simulink model "sampleModel1739"  (R2022a)
settings: Solver=FixedStepAuto  StartTime=0.0  StopTime=10.0  RelTol=1e-3
undefined symbols (not defined in the file): DiscIntNeverNeededParam, Newton, Raphson
libraries: simulink x34, slpidlib x7
(part 1 of 2)
settings Model: SimulationMode=software-in-the-loop (sil)  Creator=lenovo  LastModifiedBy=TSMC
settings DataIOCC: InspectSignalLogs=on  SignalLoggingName=logsOut
settings OptimizationCC: DefaultParameterBehavior=Inlined  EnhancedBackFolding=on  PassReuseOutputArgsAs=Individual arguments  ZeroExternalMemoryAtStartup=off  ZeroInternalMemoryAtStartup=off  OptimizeBlockOrder=speed  DifferentSizesBufferReuse=on  OptimizationCustomize=off  EfficientTunableParamExpr=on
settings DebuggingCC: ParameterTunabilityLossMsg=error  UnconnectedInputMsg=warning  UnconnectedOutputMsg=warning  UnconnectedLineMsg=warning
settings ModelReferenceCC: UpdateModelReferenceTargets=Force
settings SFSimCC: MATLABDynamicMemAlloc=off
settings RTWCC: SystemTargetFile=ert.tlc  TemplateMakefile=ert_default_tmf  GenerateReport=on  IncludeHyperlinkInReport=on  GenerateTraceInfo=on  DLArmComputeVersion=19.05
settings CodeAppCC: ForceParamTrailComments=on  IgnoreCustomStorageClasses=off  OperatorAnnotations=on  SimulinkDataObjDesc=on  SFDataObjDesc=on  InsertBlockDesc=on
settings ERTTargetCC: TargetLangStandard=C99 (ISO)  GenerateSampleERTMain=on  SupportContinuousTime=on  InlinedParameterPlacement=NonHierarchical  ERTCustomFileTemplate=example_file_process.tlc

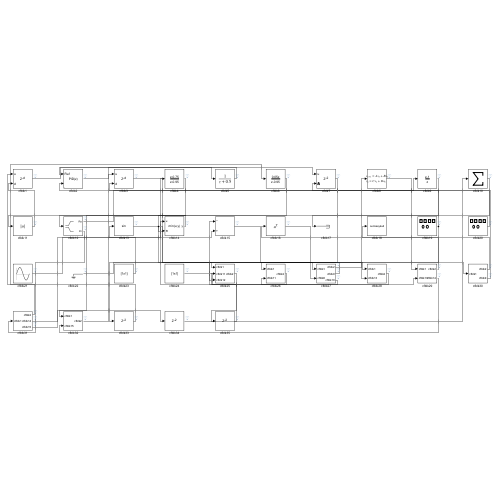
[thumbnail: Simulink's stored preview of the top-level diagram]
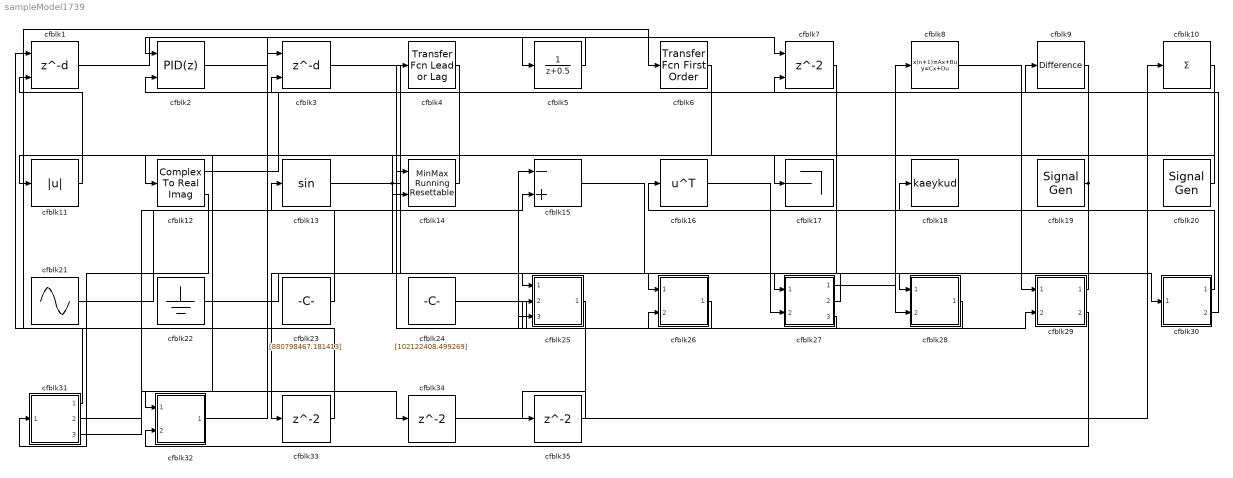
== system sampleModel1739 ==
  cfblk1 : Delay  DelayLengthSource=Input port  SampleTime=1
      settings: InputPortMap=u0,p1
  cfblk10 : Sum  Inputs=+
  cfblk11 : Abs  SaturateOnIntegerOverflow=off
  cfblk12 : ComplexToRealImag
  cfblk13 : Trigonometry
  cfblk14 : simulink/Math Operations/MinMax Running Resettable  Function=min  vinit=0.0
  cfblk15 : Sum  Inputs=-+
  cfblk16 : Math  Operator=transpose
  cfblk17 : Terminator
  cfblk18 : ToWorkspace  VariableName=kaeykud  SaveFormat=Timeseries  SampleTime=-1
  cfblk19 : SignalGenerator  WaveForm=sawtooth  Amplitude=[-934882959.011035]  Units=rad/sec
  cfblk2 : slpidlib/PID Controller (2DOF)  Controller=PID  Form=Parallel  TimeDomain=Discrete-time  UseExternalTs=off  SampleTime=1  IntegratorMethod=Forward Euler  FilterMethod=Forward Euler  ControllerParametersSource=internal  P=1  I=1  UseKiTs=off  D=0  N=100  UseFilter=on  b=1  c=1  TunerSelectOption=Transfer Function Based (PID Tuner App)  InitialConditionSource=internal  InitialConditionForIntegrator=0  InitialConditionForFilter=0  DifferentiatorICPrevScaledInput=0  ExternalReset=none  TrackingMode=off  Kt=1  LimitOutput=off  SatLimitsSource=internal  UpperSaturationLimit=inf  LowerSaturationLimit=-inf  LinearizeAsGain=off  AntiWindupMode=none  Kb=1  POutMin=[]  POutMax=[]  IOutMin=[]  IOutMax=[]  DOutMin=[]  DOutMax=[]  NOutMin=[]  NOutMax=[]  bOutMin=[]  bOutMax=[]  cOutMin=[]  cOutMax=[]  SumOutMin=[]  SumOutMax=[]  SaturationOutMin=[]  SaturationOutMax=[]  PParamMin=[]  PParamMax=[]  IParamMin=[]  IParamMax=[]  DParamMin=[]  DParamMax=[]  NParamMin=[]  NParamMax=[]  bParamMin=[]  bParamMax=[]  cParamMin=[]  cParamMax=[]  KbParamMin=[]  KbParamMax=[]  KtParamMin=[]  KtParamMax=[]  KbOutMin=[]  KbOutMax=[]  KtOutMin=[]  KtOutMax=[]  IntegratorOutMin=[]  IntegratorOutMax=[]  FilterOutMin=[]  FilterOutMax=[]  SumI1OutMin=[]  SumI1OutMax=[]  SumI2OutMin=[]  SumI2OutMax=[]  SumI3OutMin=[]  SumI3OutMax=[]  SumI4OutMin=[]  SumI4OutMax=[]  SumDOutMin=[]  SumDOutMax=[]  Sum1OutMin=[]  Sum1OutMax=[]  Sum2OutMin=[]  Sum2OutMax=[]  Sum3OutMin=[]  Sum3OutMax=[]  DifferentiatorOutMin=[]  DifferentiatorOutMax=[]  FilterDiffOutCoefMin=[]  FilterDiffOutCoefMax=[]  ReciprocalOutMin=[]  ReciprocalOutMax=[]  SumDenOutMin=[]  SumDenOutMax=[]  SumNumOutMin=[]  SumNumOutMax=[]  DivideOutMin=[]  DivideOutMax=[]  UdiffTsProdOutMin=[]  UdiffTsProdOutMax=[]  NTsProdOutMin=[]  NTsProdOutMax=[]  UintegralTsProdOutMin=[]  UintegralTsProdOutMax=[]  UngainTsProdOutMin=[]  UngainTsProdOutMax=[]  IntegratorContinuousStateAttributes=''  IntegratorStateMustResolveToSignalObject=off  IntegratorRTWStateStorageClass=Auto  FilterContinuousStateAttributes=''  FilterStateMustResolveToSignalObject=off  FilterRTWStateStorageClass=Auto  ParallelPVariant=InternalParameters  IdealPVariant=Disabled  IVariant=InternalParameters  DVariant=InternalParameters  bVariant=InternalParameters  cVariant=InternalParameters  IntegratorVariant=Discrete  SatVariant=Disabled  AWVariant=Passthrough  PCopyVariant=Disabled  TRVariant=Disabled  FdbkBlocksVariant=Forward  IdealPFdbkVariant=Disabled  SatFdbkVariant=Disabled  DerivativeFilterVariant=ForwardEulerFilter  NVariant=InternalParameters  NCopyVariant=Disabled  FilterICVariant=InternalICsFilter  IntegratorICVariant=InternalICs  ExternalResetVariant=Disabled  TRSumVariant=Passthrough  SumFdbkVariant=Disabled  SumVariant=Sum_PID  TsampFilterVariant=InternalTs  TsampNgainVariant=Passthrough  TsampIntegralVariant=Passthrough  ExternalSaturationOutDataTypeStr=Inherit: Same as second input
      settings: SourceProductBaseCode=SL
  cfblk20 : SignalGenerator  WaveForm=square  Amplitude=[-890295358.214809]
  cfblk21 : Sin  Amplitude=[-919056267.570477]  Bias=[51069111.724816]  SampleTime=0
  cfblk22 : Ground
  cfblk23 : Constant  Value=[880798467.181413]  SampleTime=1
  cfblk24 : Constant  Value=[102122408.499269]  SampleTime=1
  cfblk25 : Subsystem
  cfblk26 : Subsystem
  cfblk27 : Subsystem
  cfblk28 : Subsystem
  cfblk29 : Subsystem
  cfblk3 : Delay  DelayLengthSource=Input port  SampleTime=1
      settings: InputPortMap=u0,p1
  cfblk30 : Subsystem
  cfblk31 : Subsystem
  cfblk32 : Subsystem
  cfblk33 : Delay  SampleTime=1
  cfblk34 : Delay  SampleTime=1
  cfblk35 : Delay  SampleTime=1
  cfblk4 : simulink/Discrete/Transfer Fcn Lead or Lag  PoleZ=0.95  ZeroZ=0.75  ICPrevOutput=0.0  ICPrevInput=0.0  DoSatur=off
      settings: SourceProductBaseCode=SL
  cfblk5 : DiscreteTransferFcn  SampleTime=1
  cfblk6 : simulink/Discrete/Transfer Fcn First Order  PoleZ=0.95  ICPrevOutput=0.0  DoSatur=off
  cfblk7 : Delay  ShowEnablePort=on  SampleTime=1
      settings: InputPortMap=u0,e6
  cfblk8 : DiscreteStateSpace
  cfblk9 : simulink/Discrete/Difference  ICPrevInput=0.0  OutMin=[]  OutMax=[]  OutDataTypeStr=Inherit: Inherit via back propagation  OutDataType=fixdt(1, 16)  OutScaling=2^-10  DoSatur=off
  wires:
  cfblk30/1(cfblk2) -> cfblk16/1
  cfblk1/1 -> cfblk5/1
  cfblk3/1 -> cfblk30/1(cfblk1)
  cfblk28/1(cfblk2) -> cfblk4/1
  cfblk15/1 -> cfblk27/1(cfblk1)
  cfblk31/1(cfblk2) -> cfblk6/1
  cfblk14/1 -> cfblk12/1
  cfblk23/1 -> cfblk13/1
  cfblk4/1 -> cfblk11/1
  cfblk32/1(cfblk2) -> cfblk3/1
  cfblk13/1 -> cfblk27/2(cfblk8), cfblk28/2(cfblk13)
  cfblk12/1 -> cfblk9/1
  cfblk8/1 -> cfblk29/1(cfblk1)
  cfblk24/1 -> cfblk29/2(cfblk13)
  cfblk12/2 -> cfblk31/1(cfblk1)
  cfblk2/1 -> cfblk7/1
  cfblk9/1 -> cfblk17/1
  cfblk20/1 -> cfblk3/2
  cfblk6/1 -> cfblk32/1(cfblk1)
  cfblk11/1 -> cfblk1/2
  cfblk21/1 -> cfblk14/1
  cfblk5/1 -> cfblk2/1
  cfblk29/1(cfblk2) -> cfblk18/1
  cfblk19/1 -> cfblk2/2, cfblk25/3(cfblk12)
  cfblk31/3(cfblk15) -> cfblk15/2
  cfblk30/2(cfblk9) -> cfblk7/2
  cfblk27/1(cfblk2) -> cfblk8/1
  cfblk10/1 -> cfblk14/2
  cfblk16/1 -> cfblk28/1(cfblk1)
  cfblk22/1 -> cfblk25/1(cfblk1)
  cfblk29/2(cfblk14) -> cfblk32/2(cfblk15)
  cfblk27/2(cfblk9) -> cfblk26/1(cfblk1)
  cfblk27/3(cfblk10) -> cfblk26/2(cfblk11)
  cfblk26/1(cfblk2) -> cfblk25/2(cfblk11)
  cfblk7/1 -> cfblk33/1
  cfblk33/1 -> cfblk1/1
  cfblk31/2(cfblk14) -> cfblk34/1
  cfblk34/1 -> cfblk10/1
  cfblk25/1(cfblk2) -> cfblk35/1
  cfblk35/1 -> cfblk15/1

== system sampleModel1739/cfblk25 ==
  cfblk1 : Inport
  cfblk11 : Inport  Port=2
  cfblk12 : Inport  Port=3
  cfblk10 : Subsystem
  cfblk13 : Delay  SampleTime=1
  cfblk14 : Delay  SampleTime=1
  cfblk3 : simulink/Discrete/Tapped Delay  vinit=0.0  samptime=-1  NumDelays=1  DelayOrder=Oldest  includeCurrent=off
  cfblk4 : Signum
  cfblk5 : Sum
  cfblk6 : Sum  Inputs=+
  cfblk7 : Assignment  DiagnosticForDimensions=Warning  IndexOptions=Index vector (dialog)  Indices=1  OutputSizes=1
  cfblk8 : Constant  Value=[-767685989.889519]  SampleTime=1
  cfblk9 : Subsystem
  cfblk2 : Outport
  wires:
  cfblk10/1(cfblk2) -> cfblk9/1(cfblk1)
  cfblk8/1 -> cfblk3/1
  cfblk12/1 -> cfblk7/1
  cfblk4/1 -> cfblk10/2(cfblk14), cfblk9/4(cfblk9)
  cfblk11/1 -> cfblk10/3(cfblk15)
  cfblk10/2(cfblk17) -> cfblk9/2(cfblk7)
  cfblk5/1 -> cfblk7/2
  cfblk6/1 -> cfblk10/4(cfblk16), cfblk5/1
  cfblk1/1 -> cfblk2/1
  cfblk3/1 -> cfblk6/1, cfblk9/3(cfblk8)
  cfblk7/1 -> cfblk4/1, cfblk14/1
  cfblk9/1(cfblk2) -> cfblk13/1
  cfblk13/1 -> cfblk10/1(cfblk1)
  cfblk14/1 -> cfblk5/2

== system sampleModel1739/cfblk26 ==
  cfblk1 : Inport
  cfblk11 : Inport  Port=2
  cfblk10 : Subsystem
  cfblk12 : Delay  SampleTime=1
  cfblk3 : simulink/Discrete/Transfer Fcn First Order  PoleZ=0.95  ICPrevOutput=0.0  DoSatur=off
  cfblk4 : Sum  Inputs=|++
  cfblk5 : MinMax  Function=max  Inputs=2
  cfblk6 : Sin  TimeSource=Use external signal  SampleTime=0
  cfblk7 : Signum
  cfblk8 : Subsystem
  cfblk9 : Subsystem
  cfblk2 : Outport
  wires:
  cfblk4/1 -> cfblk7/1
  cfblk3/1 -> cfblk4/1, cfblk5/1
  cfblk1/1 -> cfblk10/1(cfblk1)
  cfblk8/1(cfblk2) -> cfblk9/1(cfblk1)
  cfblk11/1 -> cfblk4/2, cfblk8/1(cfblk1)
  cfblk9/1(cfblk2) -> cfblk10/2(cfblk6)
  cfblk10/1(cfblk2) -> cfblk6/1
  cfblk6/1 -> cfblk2/1
  cfblk7/1 -> cfblk9/2(cfblk8), cfblk9/3(cfblk9)
  cfblk9/2(cfblk10) -> cfblk10/3(cfblk7), cfblk5/2
  cfblk5/1 -> cfblk12/1
  cfblk12/1 -> cfblk3/1

== system sampleModel1739/cfblk27 ==
  cfblk1 : Inport
  cfblk8 : Inport  Port=2
  cfblk11 : Delay  SampleTime=1
  cfblk3 : Delay  SampleTime=1
  cfblk4 : DiscreteFilter  SampleTime=1
  cfblk5 : Bias  Bias=[214657201.126867]  SaturateOnIntegerOverflow=off
  cfblk6 : Constant  Value=[682272621.447085]  SampleTime=1
  cfblk7 : Subsystem
  cfblk2 : Outport
  cfblk9 : Outport  Port=2
  cfblk10 : Outport  Port=3
  wires:
  cfblk1/1 -> cfblk2/1
  cfblk8/1 -> cfblk3/1, cfblk7/2(cfblk10)
  cfblk3/1 -> cfblk10/1
  cfblk5/1 -> cfblk4/1, cfblk7/3(cfblk11)
  cfblk4/1 -> cfblk9/1
  cfblk6/1 -> cfblk7/1(cfblk1), cfblk7/4(cfblk12), cfblk7/5(cfblk13)
  cfblk7/1(cfblk2) -> cfblk11/1
  cfblk11/1 -> cfblk5/1

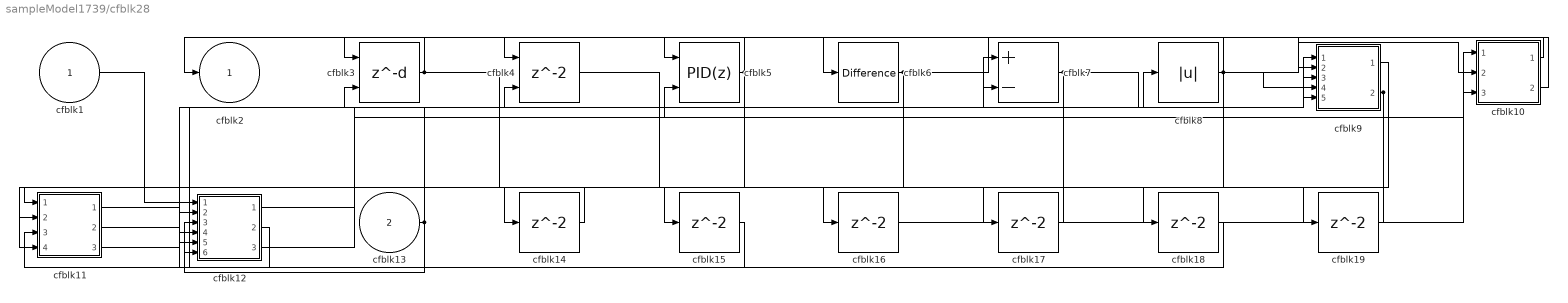
== system sampleModel1739/cfblk28 ==
  cfblk1 : Inport
  cfblk13 : Inport  Port=2
  cfblk10 : Subsystem
  cfblk11 : Subsystem
  cfblk12 : Subsystem
  cfblk{14..19} (6 alike) : Delay  SampleTime=1
  cfblk3 : Delay  DelayLengthSource=Input port  SampleTime=1
      settings: InputPortMap=u0,p1
  cfblk4 : Delay  ShowEnablePort=on  SampleTime=1
      settings: InputPortMap=u0,e6
  cfblk5 : slpidlib/PID Controller (2DOF)  Controller=PID  Form=Parallel  TimeDomain=Discrete-time  UseExternalTs=off  SampleTime=1  IntegratorMethod=Forward Euler  FilterMethod=Forward Euler  ControllerParametersSource=internal  P=1  I=1  UseKiTs=off  D=0  N=100  UseFilter=on  b=1  c=1  TunerSelectOption=Transfer Function Based (PID Tuner App)  InitialConditionSource=internal  InitialConditionForIntegrator=0  InitialConditionForFilter=0  DifferentiatorICPrevScaledInput=0  ExternalReset=none  TrackingMode=off  Kt=1  LimitOutput=off  SatLimitsSource=internal  UpperSaturationLimit=inf  LowerSaturationLimit=-inf  LinearizeAsGain=off  AntiWindupMode=none  Kb=1  POutMin=[]  POutMax=[]  IOutMin=[]  IOutMax=[]  DOutMin=[]  DOutMax=[]  NOutMin=[]  NOutMax=[]  bOutMin=[]  bOutMax=[]  cOutMin=[]  cOutMax=[]  SumOutMin=[]  SumOutMax=[]  SaturationOutMin=[]  SaturationOutMax=[]  PParamMin=[]  PParamMax=[]  IParamMin=[]  IParamMax=[]  DParamMin=[]  DParamMax=[]  NParamMin=[]  NParamMax=[]  bParamMin=[]  bParamMax=[]  cParamMin=[]  cParamMax=[]  KbParamMin=[]  KbParamMax=[]  KtParamMin=[]  KtParamMax=[]  KbOutMin=[]  KbOutMax=[]  KtOutMin=[]  KtOutMax=[]  IntegratorOutMin=[]  IntegratorOutMax=[]  FilterOutMin=[]  FilterOutMax=[]  SumI1OutMin=[]  SumI1OutMax=[]  SumI2OutMin=[]  SumI2OutMax=[]  SumI3OutMin=[]  SumI3OutMax=[]  SumI4OutMin=[]  SumI4OutMax=[]  SumDOutMin=[]  SumDOutMax=[]  Sum1OutMin=[]  Sum1OutMax=[]  Sum2OutMin=[]  Sum2OutMax=[]  Sum3OutMin=[]  Sum3OutMax=[]  DifferentiatorOutMin=[]  DifferentiatorOutMax=[]  FilterDiffOutCoefMin=[]  FilterDiffOutCoefMax=[]  ReciprocalOutMin=[]  ReciprocalOutMax=[]  SumDenOutMin=[]  SumDenOutMax=[]  SumNumOutMin=[]  SumNumOutMax=[]  DivideOutMin=[]  DivideOutMax=[]  UdiffTsProdOutMin=[]  UdiffTsProdOutMax=[]  NTsProdOutMin=[]  NTsProdOutMax=[]  UintegralTsProdOutMin=[]  UintegralTsProdOutMax=[]  UngainTsProdOutMin=[]  UngainTsProdOutMax=[]  IntegratorContinuousStateAttributes=''  IntegratorStateMustResolveToSignalObject=off  IntegratorRTWStateStorageClass=Auto  FilterContinuousStateAttributes=''  FilterStateMustResolveToSignalObject=off  FilterRTWStateStorageClass=Auto  ParallelPVariant=InternalParameters  IdealPVariant=Disabled  IVariant=InternalParameters  DVariant=InternalParameters  bVariant=InternalParameters  cVariant=InternalParameters  IntegratorVariant=Discrete  SatVariant=Disabled  AWVariant=Passthrough  PCopyVariant=Disabled  TRVariant=Disabled  FdbkBlocksVariant=Forward  IdealPFdbkVariant=Disabled  SatFdbkVariant=Disabled  DerivativeFilterVariant=ForwardEulerFilter  NVariant=InternalParameters  NCopyVariant=Disabled  FilterICVariant=InternalICsFilter  IntegratorICVariant=InternalICs  ExternalResetVariant=Disabled  TRSumVariant=Passthrough  SumFdbkVariant=Disabled  SumVariant=Sum_PID  TsampFilterVariant=InternalTs  TsampNgainVariant=Passthrough  TsampIntegralVariant=Passthrough  ExternalSaturationOutDataTypeStr=Inherit: Same as second input
      settings: SourceProductBaseCode=SL
  cfblk6 : simulink/Discrete/Difference  ICPrevInput=0.0  OutMin=[]  OutMax=[]  OutDataTypeStr=Inherit: Inherit via back propagation  OutDataType=fixdt(1, 16)  OutScaling=2^-10  DoSatur=off
  cfblk7 : Sum  Inputs=+-
  cfblk8 : Abs  SaturateOnIntegerOverflow=off
  cfblk9 : Subsystem
  cfblk2 : Outport
  wires:
  cfblk10/1(cfblk2) -> cfblk6/1
  cfblk12/1(cfblk2) -> cfblk10/1(cfblk1)
  cfblk12/2(cfblk14) -> cfblk9/1(cfblk1)
  cfblk1/1 -> cfblk12/1(cfblk1)
  cfblk3/1 -> cfblk2/1, cfblk19/1
  cfblk12/3(cfblk15) -> cfblk8/1
  cfblk13/1 -> cfblk12/3(cfblk10), cfblk3/2, cfblk11/3(cfblk10)
  cfblk5/1 -> cfblk3/1, cfblk11/2(cfblk9)
  cfblk7/1 -> cfblk9/5(cfblk12), cfblk17/1
  cfblk6/1 -> cfblk9/2(cfblk9), cfblk11/4(cfblk11)
  cfblk8/1 -> cfblk5/1, cfblk10/2(cfblk11), cfblk7/2, cfblk11/1(cfblk1), cfblk9/4(cfblk11)
  cfblk11/1(cfblk2) -> cfblk7/1
  cfblk10/2(cfblk13) -> cfblk4/1
  cfblk9/2(cfblk13) -> cfblk15/1, cfblk16/1
  cfblk11/2(cfblk12) -> cfblk9/3(cfblk10)
  cfblk11/3(cfblk13) -> cfblk4/2
  cfblk9/1(cfblk2) -> cfblk14/1
  cfblk14/1 -> cfblk12/2(cfblk9)
  cfblk15/1 -> cfblk12/6(cfblk13)
  cfblk16/1 -> cfblk10/3(cfblk12)
  cfblk17/1 -> cfblk12/4(cfblk11)
  cfblk4/1 -> cfblk18/1
  cfblk18/1 -> cfblk12/5(cfblk12)
  cfblk19/1 -> cfblk5/2

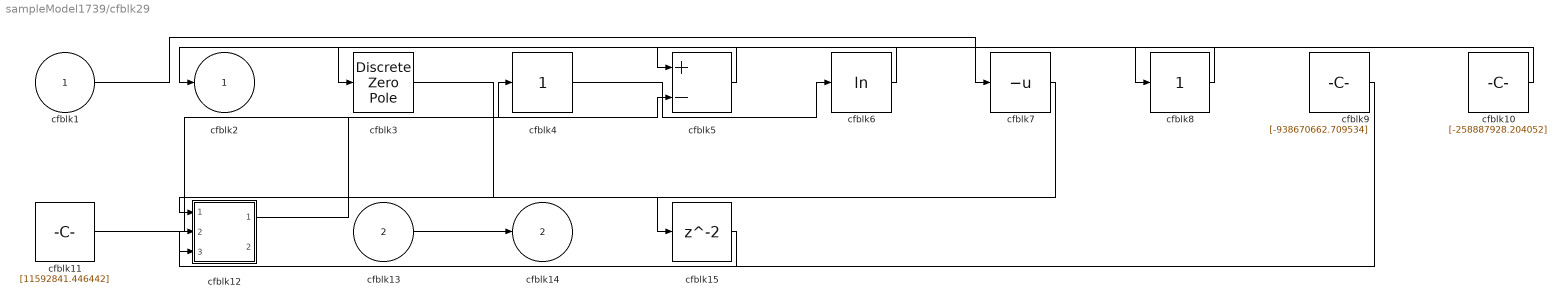
== system sampleModel1739/cfblk29 ==
  cfblk1 : Inport
  cfblk13 : Inport  Port=2
  cfblk10 : Constant  Value=[-258887928.204052]  SampleTime=1
  cfblk11 : Constant  Value=[11592841.446442]  SampleTime=1
  cfblk12 : Subsystem
  cfblk15 : Delay  SampleTime=1
  cfblk3 : DiscreteZeroPole  Poles=[0 0.5]  Gain=1
  cfblk4 : simulink/Math Operations/Slider Gain  gain=1  low=0  high=2
  cfblk5 : Sum  Inputs=+-
  cfblk6 : Math  Operator=log
  cfblk7 : UnaryMinus
  cfblk8 : simulink/Math Operations/Slider Gain  gain=1  low=0  high=2
  cfblk9 : Constant  Value=[-938670662.709534]  SampleTime=1
  cfblk2 : Outport
  cfblk14 : Outport  Port=2
  wires:
  cfblk11/1 -> cfblk4/1
  cfblk10/1 -> cfblk8/1
  cfblk6/1 -> cfblk2/1
  cfblk4/1 -> cfblk6/1
  cfblk1/1 -> cfblk7/1
  cfblk13/1 -> cfblk14/1
  cfblk5/1 -> cfblk3/1
  cfblk7/1 -> cfblk12/1(cfblk1)
  cfblk8/1 -> cfblk5/1
  cfblk9/1 -> cfblk12/2(cfblk6)
  cfblk12/1(cfblk2) -> cfblk5/2
  cfblk3/1 -> cfblk15/1
  cfblk15/1 -> cfblk12/3(cfblk7)

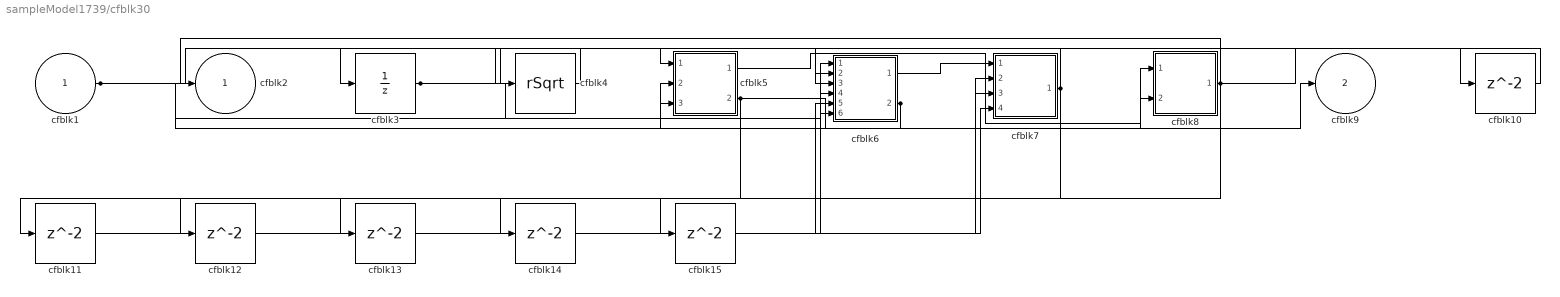
== system sampleModel1739/cfblk30 ==
  cfblk1 : Inport
  cfblk{10..15} (6 alike) : Delay  SampleTime=1
  cfblk3 : UnitDelay  HasFrameUpgradeWarning=on
  cfblk4 : Sqrt  Operator=rSqrt  AlgorithmType=Newton-Raphson
  cfblk5 : Subsystem
  cfblk6 : Subsystem
  cfblk7 : Subsystem
  cfblk8 : Subsystem
  cfblk2 : Outport
  cfblk9 : Outport  Port=2
  wires:
  cfblk7/1(cfblk2) -> cfblk5/1(cfblk1), cfblk15/1
  cfblk3/1 -> cfblk6/1(cfblk1), cfblk6/3(cfblk10)
  cfblk1/1 -> cfblk4/1, cfblk8/2(cfblk11), cfblk6/4(cfblk11)
  cfblk8/1(cfblk2) -> cfblk2/1, cfblk10/1, cfblk11/1
  cfblk5/1(cfblk2) -> cfblk8/1(cfblk1)
  cfblk5/2(cfblk15) -> cfblk9/1, cfblk12/1, cfblk13/1, cfblk14/1
  cfblk4/1 -> cfblk3/1
  cfblk6/1(cfblk2) -> cfblk7/1(cfblk1)
  cfblk6/2(cfblk14) -> cfblk5/2(cfblk13), cfblk5/3(cfblk14)
  cfblk10/1 -> cfblk6/2(cfblk9)
  cfblk11/1 -> cfblk6/6(cfblk13)
  cfblk12/1 -> cfblk7/2(cfblk13)
  cfblk13/1 -> cfblk7/3(cfblk14)
  cfblk14/1 -> cfblk7/4(cfblk15)
  cfblk15/1 -> cfblk6/5(cfblk12)

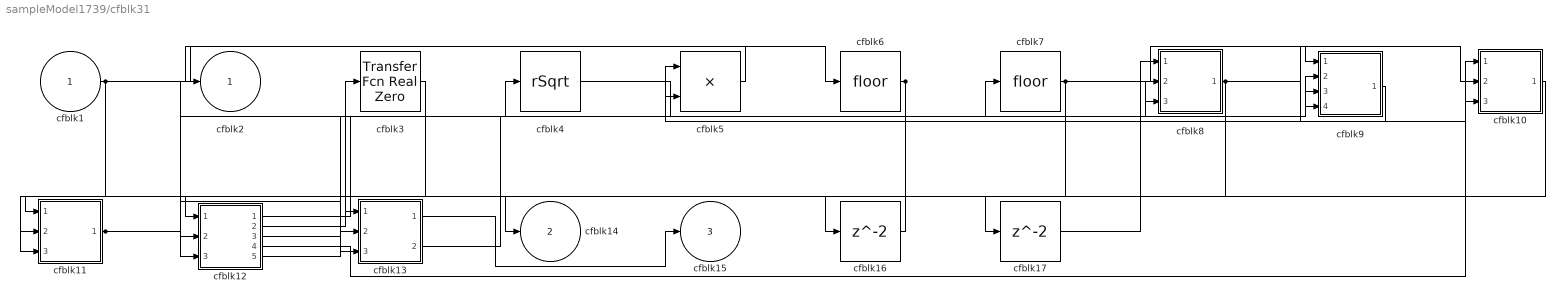
== system sampleModel1739/cfblk31 ==
  cfblk1 : Inport
  cfblk10 : Subsystem
  cfblk11 : Subsystem
  cfblk12 : Subsystem
  cfblk13 : Subsystem
  cfblk16 : Delay  SampleTime=1
  cfblk17 : Delay  SampleTime=1
  cfblk3 : simulink/Discrete/Transfer Fcn Real Zero  ZeroZ=0.75  ICPrevInput=0.0  DoSatur=off
      settings: SourceProductBaseCode=SL
  cfblk4 : Sqrt  Operator=rSqrt  AlgorithmType=Newton-Raphson
  cfblk5 : Product  Inputs=**
  cfblk6 : Rounding
  cfblk7 : Rounding
  cfblk8 : Subsystem
  cfblk9 : Subsystem
  cfblk2 : Outport
  cfblk14 : Outport  Port=2
  cfblk15 : Outport  Port=3
  wires:
  cfblk1/1 -> cfblk6/1, cfblk5/2, cfblk11/3(cfblk16), cfblk8/3(cfblk10)
  cfblk9/1(cfblk2) -> cfblk5/1
  cfblk7/1 -> cfblk9/1(cfblk1), cfblk11/1(cfblk1), cfblk11/2(cfblk15)
  cfblk6/1 -> cfblk14/1, cfblk12/2(cfblk9), cfblk12/3(cfblk10)
  cfblk12/1(cfblk2) -> cfblk7/1
  cfblk12/2(cfblk11) -> cfblk3/1
  cfblk3/1 -> cfblk13/1(cfblk1)
  cfblk13/1(cfblk2) -> cfblk15/1
  cfblk11/1(cfblk2) -> cfblk13/2(cfblk10), cfblk8/2(cfblk9), cfblk16/1
  cfblk5/1 -> cfblk2/1
  cfblk12/3(cfblk12) -> cfblk9/2(cfblk6)
  cfblk13/2(cfblk12) -> cfblk9/3(cfblk7)
  cfblk12/4(cfblk13) -> cfblk10/1(cfblk1)
  cfblk8/1(cfblk2) -> cfblk10/2(cfblk12), cfblk13/3(cfblk11), cfblk10/3(cfblk13)
  cfblk12/5(cfblk14) -> cfblk4/1
  cfblk4/1 -> cfblk9/4(cfblk8)
  cfblk16/1 -> cfblk12/1(cfblk1)
  cfblk10/1(cfblk2) -> cfblk17/1
  cfblk17/1 -> cfblk8/1(cfblk1)

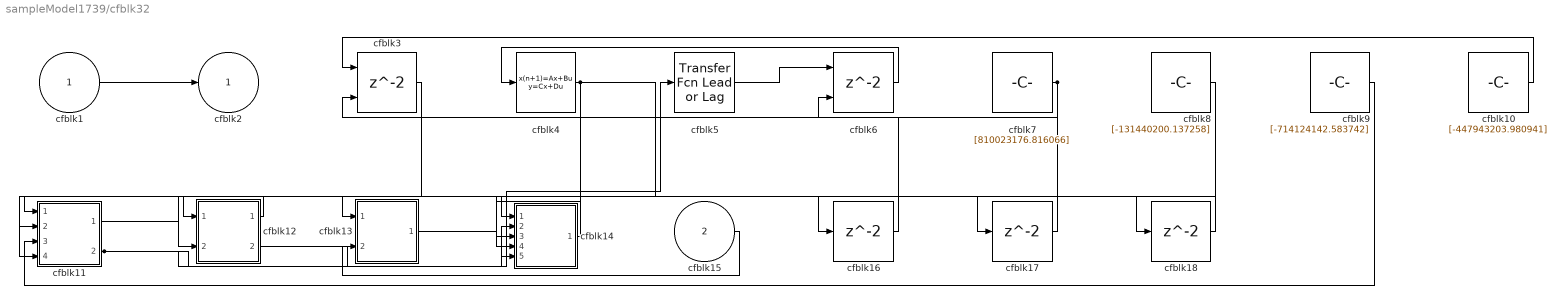
== system sampleModel1739/cfblk32 ==
  cfblk1 : Inport
  cfblk15 : Inport  Port=2
  cfblk10 : Constant  Value=[-447943203.980941]  SampleTime=1
  cfblk11 : Subsystem
  cfblk12 : Subsystem
  cfblk13 : Subsystem
  cfblk14 : Subsystem
  cfblk16 : Delay  SampleTime=1
  cfblk17 : Delay  SampleTime=1
  cfblk18 : Delay  SampleTime=1
  cfblk3 : Delay  ShowEnablePort=on  SampleTime=1
      settings: InputPortMap=u0,e6
  cfblk4 : DiscreteStateSpace
  cfblk5 : simulink/Discrete/Transfer Fcn Lead or Lag  PoleZ=0.95  ZeroZ=0.75  ICPrevOutput=0.0  ICPrevInput=0.0  DoSatur=off
      settings: SourceProductBaseCode=SL
  cfblk6 : Delay  ShowEnablePort=on  SampleTime=1
      settings: InputPortMap=u0,e6
  cfblk7 : Constant  Value=[810023176.816066]  SampleTime=1
  cfblk8 : Constant  Value=[-131440200.137258]  SampleTime=1
  cfblk9 : Constant  Value=[-714124142.583742]  SampleTime=1
  cfblk2 : Outport
  wires:
  cfblk6/1 -> cfblk4/1
  cfblk12/1(cfblk2) -> cfblk11/1(cfblk1)
  cfblk4/1 -> cfblk14/3(cfblk13), cfblk14/4(cfblk14), cfblk17/1
  cfblk10/1 -> cfblk3/1
  cfblk11/2(cfblk7) -> cfblk5/1, cfblk14/5(cfblk15)
  cfblk5/1 -> cfblk6/1
  cfblk8/1 -> cfblk14/1(cfblk1)
  cfblk7/1 -> cfblk6/2, cfblk11/4(cfblk6)
  cfblk12/2(cfblk16) -> cfblk14/2(cfblk12)
  cfblk1/1 -> cfblk2/1
  cfblk3/1 -> cfblk12/2(cfblk15)
  cfblk14/1(cfblk2) -> cfblk13/1(cfblk1)
  cfblk15/1 -> cfblk13/2(cfblk9)
  cfblk9/1 -> cfblk11/3(cfblk5)
  cfblk11/1(cfblk2) -> cfblk16/1
  cfblk16/1 -> cfblk3/2
  cfblk17/1 -> cfblk11/2(cfblk4)
  cfblk13/1(cfblk2) -> cfblk18/1
  cfblk18/1 -> cfblk12/1(cfblk1)

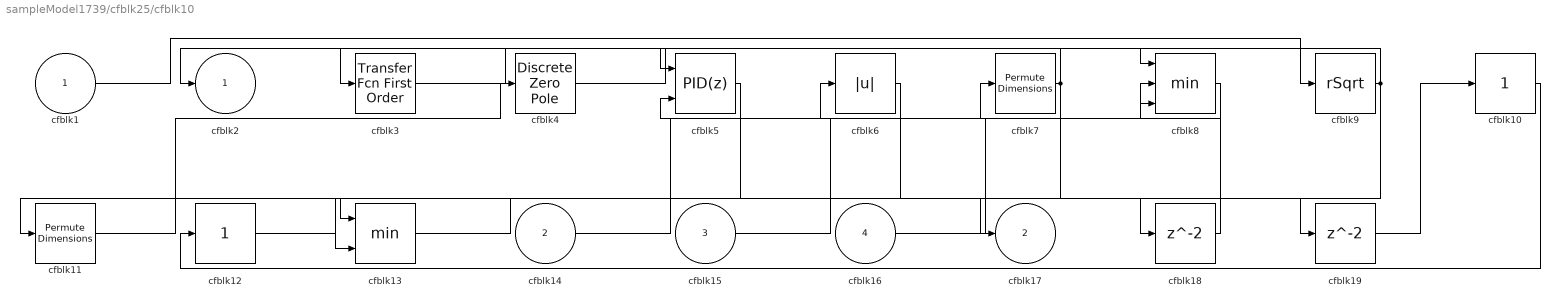
== system sampleModel1739/cfblk25/cfblk10 ==
  cfblk1 : Inport
  cfblk14 : Inport  Port=2
  cfblk15 : Inport  Port=3
  cfblk16 : Inport  Port=4
  cfblk10 : simulink/Math Operations/Slider Gain  gain=1  low=0  high=2
  cfblk11 : PermuteDimensions
  cfblk12 : simulink/Math Operations/Slider Gain  gain=1  low=0  high=2
  cfblk13 : MinMax  Inputs=2
  cfblk18 : Delay  SampleTime=1
  cfblk19 : Delay  SampleTime=1
  cfblk3 : simulink/Discrete/Transfer Fcn First Order  PoleZ=0.95  ICPrevOutput=0.0  DoSatur=off
  cfblk4 : DiscreteZeroPole  Poles=[0 0.5]  Gain=1
  cfblk5 : slpidlib/PID Controller (2DOF)  Controller=PID  Form=Parallel  TimeDomain=Discrete-time  UseExternalTs=off  SampleTime=1  IntegratorMethod=Forward Euler  FilterMethod=Forward Euler  ControllerParametersSource=internal  P=1  I=1  UseKiTs=off  D=0  N=100  UseFilter=on  b=1  c=1  TunerSelectOption=Transfer Function Based (PID Tuner App)  InitialConditionSource=internal  InitialConditionForIntegrator=0  InitialConditionForFilter=0  DifferentiatorICPrevScaledInput=0  ExternalReset=none  TrackingMode=off  Kt=1  LimitOutput=off  SatLimitsSource=internal  UpperSaturationLimit=inf  LowerSaturationLimit=-inf  LinearizeAsGain=off  AntiWindupMode=none  Kb=1  POutMin=[]  POutMax=[]  IOutMin=[]  IOutMax=[]  DOutMin=[]  DOutMax=[]  NOutMin=[]  NOutMax=[]  bOutMin=[]  bOutMax=[]  cOutMin=[]  cOutMax=[]  SumOutMin=[]  SumOutMax=[]  SaturationOutMin=[]  SaturationOutMax=[]  PParamMin=[]  PParamMax=[]  IParamMin=[]  IParamMax=[]  DParamMin=[]  DParamMax=[]  NParamMin=[]  NParamMax=[]  bParamMin=[]  bParamMax=[]  cParamMin=[]  cParamMax=[]  KbParamMin=[]  KbParamMax=[]  KtParamMin=[]  KtParamMax=[]  KbOutMin=[]  KbOutMax=[]  KtOutMin=[]  KtOutMax=[]  IntegratorOutMin=[]  IntegratorOutMax=[]  FilterOutMin=[]  FilterOutMax=[]  SumI1OutMin=[]  SumI1OutMax=[]  SumI2OutMin=[]  SumI2OutMax=[]  SumI3OutMin=[]  SumI3OutMax=[]  SumI4OutMin=[]  SumI4OutMax=[]  SumDOutMin=[]  SumDOutMax=[]  Sum1OutMin=[]  Sum1OutMax=[]  Sum2OutMin=[]  Sum2OutMax=[]  Sum3OutMin=[]  Sum3OutMax=[]  DifferentiatorOutMin=[]  DifferentiatorOutMax=[]  FilterDiffOutCoefMin=[]  FilterDiffOutCoefMax=[]  ReciprocalOutMin=[]  ReciprocalOutMax=[]  SumDenOutMin=[]  SumDenOutMax=[]  SumNumOutMin=[]  SumNumOutMax=[]  DivideOutMin=[]  DivideOutMax=[]  UdiffTsProdOutMin=[]  UdiffTsProdOutMax=[]  NTsProdOutMin=[]  NTsProdOutMax=[]  UintegralTsProdOutMin=[]  UintegralTsProdOutMax=[]  UngainTsProdOutMin=[]  UngainTsProdOutMax=[]  IntegratorContinuousStateAttributes=''  IntegratorStateMustResolveToSignalObject=off  IntegratorRTWStateStorageClass=Auto  FilterContinuousStateAttributes=''  FilterStateMustResolveToSignalObject=off  FilterRTWStateStorageClass=Auto  ParallelPVariant=InternalParameters  IdealPVariant=Disabled  IVariant=InternalParameters  DVariant=InternalParameters  bVariant=InternalParameters  cVariant=InternalParameters  IntegratorVariant=Discrete  SatVariant=Disabled  AWVariant=Passthrough  PCopyVariant=Disabled  TRVariant=Disabled  FdbkBlocksVariant=Forward  IdealPFdbkVariant=Disabled  SatFdbkVariant=Disabled  DerivativeFilterVariant=ForwardEulerFilter  NVariant=InternalParameters  NCopyVariant=Disabled  FilterICVariant=InternalICsFilter  IntegratorICVariant=InternalICs  ExternalResetVariant=Disabled  TRSumVariant=Passthrough  SumFdbkVariant=Disabled  SumVariant=Sum_PID  TsampFilterVariant=InternalTs  TsampNgainVariant=Passthrough  TsampIntegralVariant=Passthrough  ExternalSaturationOutDataTypeStr=Inherit: Same as second input
      settings: SourceProductBaseCode=SL
  cfblk6 : Abs  SaturateOnIntegerOverflow=off
  cfblk7 : PermuteDimensions
  cfblk8 : MinMax  Inputs=3
  cfblk9 : Sqrt  Operator=rSqrt  AlgorithmType=Newton-Raphson
  cfblk2 : Outport
  cfblk17 : Outport  Port=2
  wires:
  cfblk6/1 -> cfblk11/1
  cfblk14/1 -> cfblk6/1
  cfblk5/1 -> cfblk13/1
  cfblk4/1 -> cfblk8/1
  cfblk10/1 -> cfblk12/1
  cfblk8/1 -> cfblk7/1
  cfblk3/1 -> cfblk5/1
  cfblk7/1 -> cfblk2/1, cfblk13/2
  cfblk16/1 -> cfblk8/2
  cfblk15/1 -> cfblk8/3
  cfblk1/1 -> cfblk9/1
  cfblk9/1 -> cfblk3/1, cfblk17/1
  cfblk11/1 -> cfblk4/1
  cfblk13/1 -> cfblk18/1
  cfblk18/1 -> cfblk5/2
  cfblk12/1 -> cfblk19/1
  cfblk19/1 -> cfblk10/1

== system sampleModel1739/cfblk25/cfblk9 ==
  cfblk1 : Inport
  cfblk7 : Inport  Port=2
  cfblk8 : Inport  Port=3
  cfblk9 : Inport  Port=4
  cfblk10 : Delay  SampleTime=1
  cfblk3 : Delay  ShowEnablePort=on  SampleTime=1
      settings: InputPortMap=u0,e6
  cfblk4 : Product  Inputs=**
  cfblk5 : Squeeze
  cfblk6 : Rounding
  cfblk2 : Outport
  wires:
  cfblk3/1 -> cfblk5/1
  cfblk6/1 -> cfblk3/2
  cfblk9/1 -> cfblk4/1
  cfblk7/1 -> cfblk4/2
  cfblk4/1 -> cfblk6/1
  cfblk8/1 -> cfblk2/1
  cfblk5/1 -> cfblk10/1
  cfblk10/1 -> cfblk3/1

== system sampleModel1739/cfblk26/cfblk10 ==
  cfblk1 : Inport
  cfblk6 : Inport  Port=2
  cfblk7 : Inport  Port=3
  cfblk3 : Delay  SampleTime=1
  cfblk4 : Sum  Inputs=+-
  cfblk5 : Reshape
  cfblk2 : Outport
  wires:
  cfblk3/1 -> cfblk2/1
  cfblk1/1 -> cfblk5/1
  cfblk4/1 -> cfblk3/1
  cfblk5/1 -> cfblk4/1
  cfblk7/1 -> cfblk4/2

== system sampleModel1739/cfblk26/cfblk8 ==
  cfblk1 : Inport
  cfblk3 : Abs  SaturateOnIntegerOverflow=off
  cfblk4 : Abs  SaturateOnIntegerOverflow=off
  cfblk5 : Reshape
  cfblk6 : UnaryMinus
  cfblk7 : Sum  Inputs=+-
  cfblk8 : Constant  Value=[-331524206.150014]  SampleTime=1
  cfblk9 : Delay  SampleTime=1
  cfblk2 : Outport
  wires:
  cfblk7/1 -> cfblk3/1
  cfblk6/1 -> cfblk2/1
  cfblk4/1 -> cfblk5/1
  cfblk8/1 -> cfblk6/1
  cfblk3/1 -> cfblk4/1
  cfblk1/1 -> cfblk7/2
  cfblk5/1 -> cfblk9/1
  cfblk9/1 -> cfblk7/1

== system sampleModel1739/cfblk26/cfblk9 ==
  cfblk1 : Inport
  cfblk8 : Inport  Port=2
  cfblk9 : Inport  Port=3
  cfblk3 : ComplexToRealImag
  cfblk4 : Sum  Inputs=--
  cfblk5 : Sum  Inputs=-+
  cfblk6 : Constant  Value=[541692330.887596]  SampleTime=1
  cfblk7 : Constant  Value=[511279827.683461]  SampleTime=1
  cfblk2 : Outport
  cfblk10 : Outport  Port=2
  wires:
  cfblk9/1 -> cfblk3/1
  cfblk1/1 -> cfblk2/1
  cfblk6/1 -> cfblk5/1
  cfblk5/1 -> cfblk10/1
  cfblk3/1 -> cfblk4/1
  cfblk4/1 -> cfblk5/2
  cfblk8/1 -> cfblk4/2

== system sampleModel1739/cfblk27/cfblk7 ==
  cfblk1 : Inport
  cfblk10 : Inport  Port=2
  cfblk11 : Inport  Port=3
  cfblk12 : Inport  Port=4
  cfblk13 : Inport  Port=5
  cfblk3 : simulink/Discrete/Difference  ICPrevInput=0.0  OutMin=[]  OutMax=[]  OutDataTypeStr=Inherit: Inherit via back propagation  OutDataType=fixdt(1, 16)  OutScaling=2^-10  DoSatur=off
  cfblk4 : DiscreteFir  SampleTime=1
  cfblk5 : DiscreteFir  SampleTime=1
  cfblk6 : Assignment  DiagnosticForDimensions=Warning  IndexOptions=Index vector (dialog)  Indices=1  OutputSizes=1
  cfblk7 : MinMax  Function=max
  cfblk8 : Rounding
  cfblk9 : Constant  Value=[608619100.167560]  SampleTime=1
  cfblk2 : Outport
  wires:
  cfblk12/1 -> cfblk3/1
  cfblk3/1 -> cfblk8/1
  cfblk5/1 -> cfblk2/1
  cfblk11/1 -> cfblk6/1
  cfblk10/1 -> cfblk6/2
  cfblk8/1 -> cfblk5/1
  cfblk9/1 -> cfblk4/1
  cfblk4/1 -> cfblk7/1

== system sampleModel1739/cfblk28/cfblk10 ==
  cfblk1 : Inport
  cfblk11 : Inport  Port=2
  cfblk12 : Inport  Port=3
  cfblk10 : Constant  Value=[-961834230.043374]  SampleTime=1
  cfblk14 : Delay  SampleTime=1
  cfblk3 : DiscreteTransferFcn  SampleTime=1
  cfblk4 : slpidlib/PID Controller  Controller=PID  Form=Parallel  TimeDomain=Discrete-time  UseExternalTs=off  SampleTime=1  IntegratorMethod=Forward Euler  FilterMethod=Forward Euler  ControllerParametersSource=internal  P=1  I=1  UseKiTs=off  D=0  N=100  UseFilter=on  TunerSelectOption=Transfer Function Based (PID Tuner App)  InitialConditionSource=internal  InitialConditionForIntegrator=0  InitialConditionForFilter=0  DifferentiatorICPrevScaledInput=0  ExternalReset=none  TrackingMode=off  Kt=1  LimitOutput=off  SatLimitsSource=internal  UpperSaturationLimit=inf  LowerSaturationLimit=-inf  LinearizeAsGain=off  AntiWindupMode=none  Kb=1  POutMin=[]  POutMax=[]  IOutMin=[]  IOutMax=[]  DOutMin=[]  DOutMax=[]  NOutMin=[]  NOutMax=[]  SumOutMin=[]  SumOutMax=[]  SaturationOutMin=[]  SaturationOutMax=[]  PParamMin=[]  PParamMax=[]  IParamMin=[]  IParamMax=[]  DParamMin=[]  DParamMax=[]  NParamMin=[]  NParamMax=[]  KbParamMin=[]  KbParamMax=[]  KtParamMin=[]  KtParamMax=[]  KbOutMin=[]  KbOutMax=[]  KtOutMin=[]  KtOutMax=[]  IntegratorOutMin=[]  IntegratorOutMax=[]  FilterOutMin=[]  FilterOutMax=[]  SumI1OutMin=[]  SumI1OutMax=[]  SumI2OutMin=[]  SumI2OutMax=[]  SumI3OutMin=[]  SumI3OutMax=[]  SumI4OutMin=[]  SumI4OutMax=[]  SumDOutMin=[]  SumDOutMax=[]  DifferentiatorOutMin=[]  DifferentiatorOutMax=[]  FilterDiffOutCoefMin=[]  FilterDiffOutCoefMax=[]  ReciprocalOutMin=[]  ReciprocalOutMax=[]  SumDenOutMin=[]  SumDenOutMax=[]  SumNumOutMin=[]  SumNumOutMax=[]  DivideOutMin=[]  DivideOutMax=[]  UdiffTsProdOutMin=[]  UdiffTsProdOutMax=[]  NTsProdOutMin=[]  NTsProdOutMax=[]  UintegralTsProdOutMin=[]  UintegralTsProdOutMax=[]  UngainTsProdOutMin=[]  UngainTsProdOutMax=[]  IntegratorContinuousStateAttributes=''  IntegratorStateMustResolveToSignalObject=off  IntegratorRTWStateStorageClass=Auto  FilterContinuousStateAttributes=''  FilterStateMustResolveToSignalObject=off  FilterRTWStateStorageClass=Auto  ParallelPVariant=InternalParameters  IdealPVariant=Disabled  IVariant=InternalParameters  DVariant=InternalParameters  IntegratorVariant=Discrete  SatVariant=Disabled  AWVariant=Passthrough  PCopyVariant=Disabled  TRVariant=Disabled  FdbkBlocksVariant=Forward  IdealPFdbkVariant=Disabled  SatFdbkVariant=Disabled  DerivativeFilterVariant=ForwardEulerFilter  NVariant=InternalParameters  NCopyVariant=Disabled  FilterICVariant=InternalICsFilter  IntegratorICVariant=InternalICs  ExternalResetVariant=Disabled  TRSumVariant=Passthrough  SumFdbkVariant=Disabled  SumVariant=Sum_PID  TsampFilterVariant=InternalTs  TsampNgainVariant=Passthrough  TsampIntegralVariant=Passthrough  ExternalSaturationOutDataTypeStr=Inherit: Same as second input  aMode=0
  cfblk5 : Delay  ShowEnablePort=on  SampleTime=1
      settings: InputPortMap=u0,e6
  cfblk6 : PermuteDimensions
  cfblk7 : Product  Inputs=**
  cfblk8 : Squeeze
  cfblk9 : Sin  TimeSource=Use external signal  SampleTime=0
  cfblk2 : Outport
  cfblk13 : Outport  Port=2
  wires:
  cfblk1/1 -> cfblk9/1
  cfblk4/1 -> cfblk5/1
  cfblk10/1 -> cfblk5/2
  cfblk6/1 -> cfblk13/1
  cfblk9/1 -> cfblk2/1
  cfblk12/1 -> cfblk8/1
  cfblk8/1 -> cfblk3/1
  cfblk11/1 -> cfblk7/1
  cfblk3/1 -> cfblk6/1, cfblk7/2
  cfblk5/1 -> cfblk14/1
  cfblk14/1 -> cfblk4/1

== system sampleModel1739/cfblk28/cfblk11 ==
  cfblk1 : Inport
  cfblk9 : Inport  Port=2
  cfblk10 : Inport  Port=3
  cfblk11 : Inport  Port=4
  cfblk3 : DiscreteFilter  SampleTime=1
  cfblk4 : simulink/Discrete/Transfer Fcn First Order  PoleZ=0.95  ICPrevOutput=0.0  DoSatur=off
  cfblk5 : Product
  cfblk6 : Sum  Inputs=+-
  cfblk7 : Constant  Value=[-926436694.043455]  SampleTime=1
  cfblk8 : Constant  Value=[-858535258.577089]  SampleTime=1
  cfblk2 : Outport
  cfblk12 : Outport  Port=2
  cfblk13 : Outport  Port=3
  wires:
  cfblk10/1 -> cfblk4/1
  cfblk7/1 -> cfblk13/1
  cfblk4/1 -> cfblk6/1
  cfblk11/1 -> cfblk5/1
  cfblk9/1 -> cfblk12/1
  cfblk3/1 -> cfblk6/2
  cfblk5/1 -> cfblk2/1
  cfblk1/1 -> cfblk5/2
  cfblk8/1 -> cfblk3/1

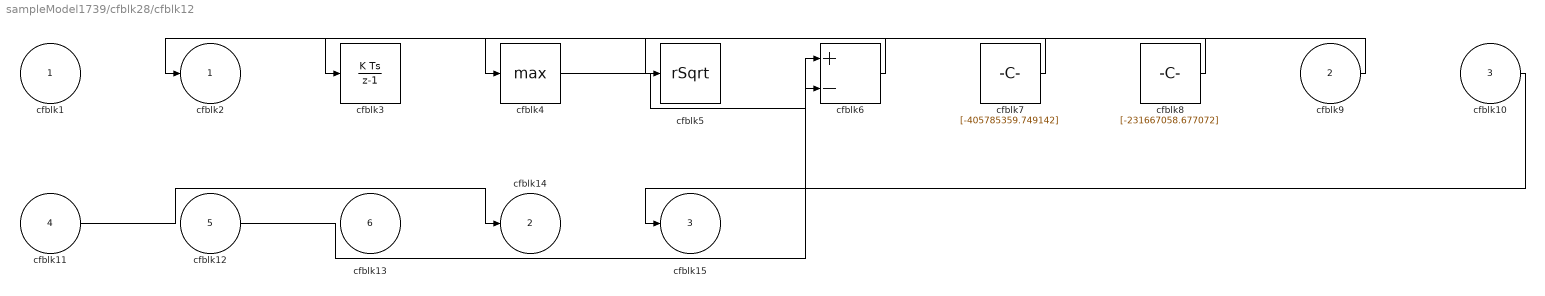
== system sampleModel1739/cfblk28/cfblk12 ==
  cfblk1 : Inport
  cfblk9 : Inport  Port=2
  cfblk10 : Inport  Port=3
  cfblk11 : Inport  Port=4
  cfblk12 : Inport  Port=5
  cfblk13 : Inport  Port=6
  cfblk3 : DiscreteIntegrator  ICPrevOutput=DiscIntNeverNeededParam  ICPrevScaledInput=DiscIntNeverNeededParam
  cfblk4 : MinMax  Function=max
  cfblk5 : Sqrt  Operator=rSqrt  AlgorithmType=Newton-Raphson
  cfblk6 : Sum  Inputs=+-
  cfblk7 : Constant  Value=[-405785359.749142]  SampleTime=1
  cfblk8 : Constant  Value=[-231667058.677072]  SampleTime=1
  cfblk2 : Outport
  cfblk14 : Outport  Port=2
  cfblk15 : Outport  Port=3
  wires:
  cfblk11/1 -> cfblk14/1
  cfblk12/1 -> cfblk6/1
  cfblk7/1 -> cfblk2/1
  cfblk4/1 -> cfblk6/2
  cfblk8/1 -> cfblk4/1
  cfblk9/1 -> cfblk3/1
  cfblk6/1 -> cfblk5/1
  cfblk10/1 -> cfblk15/1

== system sampleModel1739/cfblk28/cfblk9 ==
  cfblk1 : Inport
  cfblk9 : Inport  Port=2
  cfblk10 : Inport  Port=3
  cfblk11 : Inport  Port=4
  cfblk12 : Inport  Port=5
  cfblk14 : Delay  SampleTime=1
  cfblk3 : simulink/Discrete/Difference  ICPrevInput=0.0  OutMin=[]  OutMax=[]  OutDataTypeStr=Inherit: Inherit via back propagation  OutDataType=fixdt(1, 16)  OutScaling=2^-10  DoSatur=off
  cfblk4 : Assignment  DiagnosticForDimensions=Warning  IndexOptions=Index vector (dialog)  Indices=1  OutputSizes=1
  cfblk5 : Reshape
  cfblk6 : Trigonometry
  cfblk7 : Sum  Inputs=|++
  cfblk8 : UnaryMinus
  cfblk2 : Outport
  cfblk13 : Outport  Port=2
  wires:
  cfblk6/1 -> cfblk4/1
  cfblk4/1 -> cfblk13/1
  cfblk3/1 -> cfblk5/1
  cfblk11/1 -> cfblk7/1
  cfblk7/1 -> cfblk8/1
  cfblk9/1 -> cfblk4/2
  cfblk8/1 -> cfblk2/1
  cfblk1/1 -> cfblk7/2
  cfblk10/1 -> cfblk6/1
  cfblk5/1 -> cfblk14/1
  cfblk14/1 -> cfblk3/1

== system sampleModel1739/cfblk29/cfblk12 ==
  cfblk1 : Inport
  cfblk6 : Inport  Port=2
  cfblk7 : Inport  Port=3
  cfblk3 : Delay  DelayLengthSource=Input port  SampleTime=1
      settings: InputPortMap=u0,p1
  cfblk4 : Rounding
  cfblk5 : Math  Operator=log
  cfblk2 : Outport
  cfblk8 : Outport  Port=2
  wires:
  cfblk4/1 -> cfblk5/1
  cfblk5/1 -> cfblk8/1
  cfblk6/1 -> cfblk2/1
  cfblk1/1 -> cfblk4/1, cfblk3/2
  cfblk7/1 -> cfblk3/1

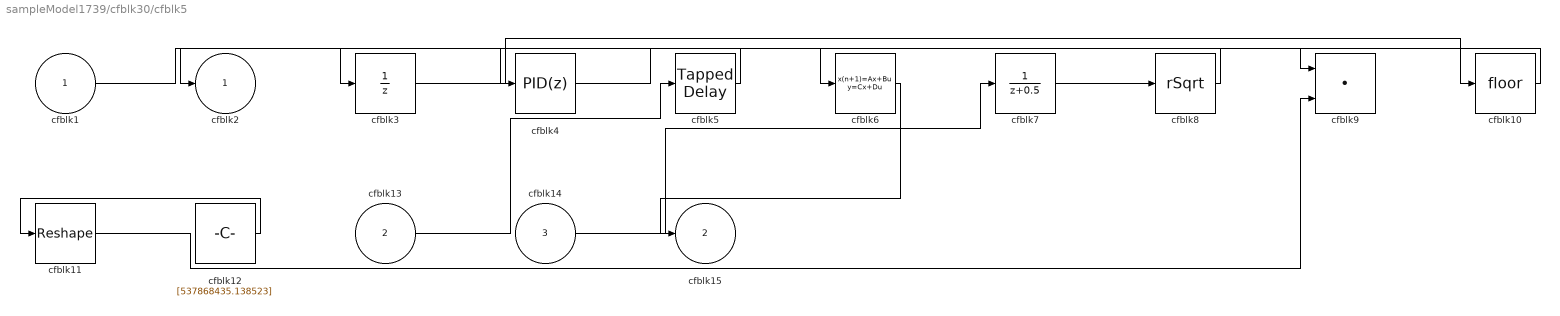
== system sampleModel1739/cfblk30/cfblk5 ==
  cfblk1 : Inport
  cfblk13 : Inport  Port=2
  cfblk14 : Inport  Port=3
  cfblk10 : Rounding
  cfblk11 : Reshape
  cfblk12 : Constant  Value=[537868435.138523]  SampleTime=1
  cfblk3 : UnitDelay  HasFrameUpgradeWarning=on
  cfblk4 : slpidlib/PID Controller  Controller=PID  Form=Parallel  TimeDomain=Discrete-time  UseExternalTs=off  SampleTime=1  IntegratorMethod=Forward Euler  FilterMethod=Forward Euler  ControllerParametersSource=internal  P=1  I=1  UseKiTs=off  D=0  N=100  UseFilter=on  TunerSelectOption=Transfer Function Based (PID Tuner App)  InitialConditionSource=internal  InitialConditionForIntegrator=0  InitialConditionForFilter=0  DifferentiatorICPrevScaledInput=0  ExternalReset=none  TrackingMode=off  Kt=1  LimitOutput=off  SatLimitsSource=internal  UpperSaturationLimit=inf  LowerSaturationLimit=-inf  LinearizeAsGain=off  AntiWindupMode=none  Kb=1  POutMin=[]  POutMax=[]  IOutMin=[]  IOutMax=[]  DOutMin=[]  DOutMax=[]  NOutMin=[]  NOutMax=[]  SumOutMin=[]  SumOutMax=[]  SaturationOutMin=[]  SaturationOutMax=[]  PParamMin=[]  PParamMax=[]  IParamMin=[]  IParamMax=[]  DParamMin=[]  DParamMax=[]  NParamMin=[]  NParamMax=[]  KbParamMin=[]  KbParamMax=[]  KtParamMin=[]  KtParamMax=[]  KbOutMin=[]  KbOutMax=[]  KtOutMin=[]  KtOutMax=[]  IntegratorOutMin=[]  IntegratorOutMax=[]  FilterOutMin=[]  FilterOutMax=[]  SumI1OutMin=[]  SumI1OutMax=[]  SumI2OutMin=[]  SumI2OutMax=[]  SumI3OutMin=[]  SumI3OutMax=[]  SumI4OutMin=[]  SumI4OutMax=[]  SumDOutMin=[]  SumDOutMax=[]  DifferentiatorOutMin=[]  DifferentiatorOutMax=[]  FilterDiffOutCoefMin=[]  FilterDiffOutCoefMax=[]  ReciprocalOutMin=[]  ReciprocalOutMax=[]  SumDenOutMin=[]  SumDenOutMax=[]  SumNumOutMin=[]  SumNumOutMax=[]  DivideOutMin=[]  DivideOutMax=[]  UdiffTsProdOutMin=[]  UdiffTsProdOutMax=[]  NTsProdOutMin=[]  NTsProdOutMax=[]  UintegralTsProdOutMin=[]  UintegralTsProdOutMax=[]  UngainTsProdOutMin=[]  UngainTsProdOutMax=[]  IntegratorContinuousStateAttributes=''  IntegratorStateMustResolveToSignalObject=off  IntegratorRTWStateStorageClass=Auto  FilterContinuousStateAttributes=''  FilterStateMustResolveToSignalObject=off  FilterRTWStateStorageClass=Auto  ParallelPVariant=InternalParameters  IdealPVariant=Disabled  IVariant=InternalParameters  DVariant=InternalParameters  IntegratorVariant=Discrete  SatVariant=Disabled  AWVariant=Passthrough  PCopyVariant=Disabled  TRVariant=Disabled  FdbkBlocksVariant=Forward  IdealPFdbkVariant=Disabled  SatFdbkVariant=Disabled  DerivativeFilterVariant=ForwardEulerFilter  NVariant=InternalParameters  NCopyVariant=Disabled  FilterICVariant=InternalICsFilter  IntegratorICVariant=InternalICs  ExternalResetVariant=Disabled  TRSumVariant=Passthrough  SumFdbkVariant=Disabled  SumVariant=Sum_PID  TsampFilterVariant=InternalTs  TsampNgainVariant=Passthrough  TsampIntegralVariant=Passthrough  ExternalSaturationOutDataTypeStr=Inherit: Same as second input  aMode=0
  cfblk5 : simulink/Discrete/Tapped Delay  vinit=0.0  samptime=-1  NumDelays=1  DelayOrder=Oldest  includeCurrent=off
  cfblk6 : DiscreteStateSpace
  cfblk7 : DiscreteTransferFcn  SampleTime=1
  cfblk8 : Sqrt  Operator=rSqrt  AlgorithmType=Newton-Raphson
  cfblk9 : DotProduct  OutDataTypeStr=Inherit: Inherit via internal rule
  cfblk2 : Outport
  cfblk15 : Outport  Port=2
  wires:
  cfblk7/1 -> cfblk8/1
  cfblk12/1 -> cfblk11/1
  cfblk13/1 -> cfblk5/1
  cfblk14/1 -> cfblk7/1
  cfblk4/1 -> cfblk9/1
  cfblk3/1 -> cfblk10/1
  cfblk5/1 -> cfblk2/1
  cfblk8/1 -> cfblk3/1
  cfblk1/1 -> cfblk6/1
  cfblk10/1 -> cfblk4/1
  cfblk11/1 -> cfblk9/2
  cfblk6/1 -> cfblk15/1

== system sampleModel1739/cfblk30/cfblk6 ==
  cfblk1 : Inport
  cfblk9 : Inport  Port=2
  cfblk10 : Inport  Port=3
  cfblk11 : Inport  Port=4
  cfblk12 : Inport  Port=5
  cfblk13 : Inport  Port=6
  cfblk15 : Delay  SampleTime=1
  cfblk3 : Delay  SampleTime=1
  cfblk4 : simulink/Math Operations/Slider Gain  gain=1  low=0  high=2
  cfblk5 : Sum  Inputs=|++
  cfblk6 : Trigonometry
  cfblk7 : MinMax  Function=max  Inputs=3
  cfblk8 : Constant  Value=[144993199.729211]  SampleTime=1
  cfblk2 : Outport
  cfblk14 : Outport  Port=2
  wires:
  cfblk6/1 -> cfblk5/1
  cfblk10/1 -> cfblk4/1
  cfblk12/1 -> cfblk6/1
  cfblk1/1 -> cfblk5/2
  cfblk4/1 -> cfblk14/1
  cfblk5/1 -> cfblk2/1
  cfblk3/1 -> cfblk7/1
  cfblk9/1 -> cfblk7/2
  cfblk11/1 -> cfblk7/3
  cfblk7/1 -> cfblk15/1
  cfblk15/1 -> cfblk3/1

== system sampleModel1739/cfblk30/cfblk7 ==
  cfblk1 : Inport
  cfblk13 : Inport  Port=2
  cfblk14 : Inport  Port=3
  cfblk15 : Inport  Port=4
  cfblk10 : Rounding
  cfblk11 : PermuteDimensions
  cfblk12 : simulink/Math Operations/MinMax Running Resettable  Function=min  vinit=0.0
  cfblk3 : Delay  SampleTime=1
  cfblk4 : DiscreteStateSpace
  cfblk5 : Reshape
  cfblk6 : Sum  Inputs=+-
  cfblk7 : Sum  Inputs=|++
  cfblk8 : Product  Inputs=*
  cfblk9 : Sum  Inputs=+-
  cfblk2 : Outport
  wires:
  cfblk5/1 -> cfblk7/1
  cfblk12/1 -> cfblk6/1
  cfblk3/1 -> cfblk10/1
  cfblk8/1 -> cfblk12/1
  cfblk7/1 -> cfblk8/1
  cfblk10/1 -> cfblk7/2
  cfblk13/1 -> cfblk6/2
  cfblk6/1 -> cfblk2/1
  cfblk1/1 -> cfblk9/1
  cfblk14/1 -> cfblk4/1
  cfblk15/1 -> cfblk11/1
  cfblk11/1 -> cfblk3/1
  cfblk4/1 -> cfblk9/2, cfblk5/1
  cfblk9/1 -> cfblk12/2

== system sampleModel1739/cfblk30/cfblk8 ==
  cfblk1 : Inport
  cfblk11 : Inport  Port=2
  cfblk10 : Assignment  DiagnosticForDimensions=Warning  IndexOptions=Index vector (dialog)  Indices=1  OutputSizes=1
  cfblk12 : Delay  SampleTime=1
  cfblk13 : Delay  SampleTime=1
  cfblk14 : Delay  SampleTime=1
  cfblk3 : simulink/Discrete/Tapped Delay  vinit=0.0  samptime=-1  NumDelays=1  DelayOrder=Oldest  includeCurrent=off
  cfblk4 : slpidlib/PID Controller (2DOF)  Controller=PID  Form=Parallel  TimeDomain=Discrete-time  UseExternalTs=off  SampleTime=1  IntegratorMethod=Forward Euler  FilterMethod=Forward Euler  ControllerParametersSource=internal  P=1  I=1  UseKiTs=off  D=0  N=100  UseFilter=on  b=1  c=1  TunerSelectOption=Transfer Function Based (PID Tuner App)  InitialConditionSource=internal  InitialConditionForIntegrator=0  InitialConditionForFilter=0  DifferentiatorICPrevScaledInput=0  ExternalReset=none  TrackingMode=off  Kt=1  LimitOutput=off  SatLimitsSource=internal  UpperSaturationLimit=inf  LowerSaturationLimit=-inf  LinearizeAsGain=off  AntiWindupMode=none  Kb=1  POutMin=[]  POutMax=[]  IOutMin=[]  IOutMax=[]  DOutMin=[]  DOutMax=[]  NOutMin=[]  NOutMax=[]  bOutMin=[]  bOutMax=[]  cOutMin=[]  cOutMax=[]  SumOutMin=[]  SumOutMax=[]  SaturationOutMin=[]  SaturationOutMax=[]  PParamMin=[]  PParamMax=[]  IParamMin=[]  IParamMax=[]  DParamMin=[]  DParamMax=[]  NParamMin=[]  NParamMax=[]  bParamMin=[]  bParamMax=[]  cParamMin=[]  cParamMax=[]  KbParamMin=[]  KbParamMax=[]  KtParamMin=[]  KtParamMax=[]  KbOutMin=[]  KbOutMax=[]  KtOutMin=[]  KtOutMax=[]  IntegratorOutMin=[]  IntegratorOutMax=[]  FilterOutMin=[]  FilterOutMax=[]  SumI1OutMin=[]  SumI1OutMax=[]  SumI2OutMin=[]  SumI2OutMax=[]  SumI3OutMin=[]  SumI3OutMax=[]  SumI4OutMin=[]  SumI4OutMax=[]  SumDOutMin=[]  SumDOutMax=[]  Sum1OutMin=[]  Sum1OutMax=[]  Sum2OutMin=[]  Sum2OutMax=[]  Sum3OutMin=[]  Sum3OutMax=[]  DifferentiatorOutMin=[]  DifferentiatorOutMax=[]  FilterDiffOutCoefMin=[]  FilterDiffOutCoefMax=[]  ReciprocalOutMin=[]  ReciprocalOutMax=[]  SumDenOutMin=[]  SumDenOutMax=[]  SumNumOutMin=[]  SumNumOutMax=[]  DivideOutMin=[]  DivideOutMax=[]  UdiffTsProdOutMin=[]  UdiffTsProdOutMax=[]  NTsProdOutMin=[]  NTsProdOutMax=[]  UintegralTsProdOutMin=[]  UintegralTsProdOutMax=[]  UngainTsProdOutMin=[]  UngainTsProdOutMax=[]  IntegratorContinuousStateAttributes=''  IntegratorStateMustResolveToSignalObject=off  IntegratorRTWStateStorageClass=Auto  FilterContinuousStateAttributes=''  FilterStateMustResolveToSignalObject=off  FilterRTWStateStorageClass=Auto  ParallelPVariant=InternalParameters  IdealPVariant=Disabled  IVariant=InternalParameters  DVariant=InternalParameters  bVariant=InternalParameters  cVariant=InternalParameters  IntegratorVariant=Discrete  SatVariant=Disabled  AWVariant=Passthrough  PCopyVariant=Disabled  TRVariant=Disabled  FdbkBlocksVariant=Forward  IdealPFdbkVariant=Disabled  SatFdbkVariant=Disabled  DerivativeFilterVariant=ForwardEulerFilter  NVariant=InternalParameters  NCopyVariant=Disabled  FilterICVariant=InternalICsFilter  IntegratorICVariant=InternalICs  ExternalResetVariant=Disabled  TRSumVariant=Passthrough  SumFdbkVariant=Disabled  SumVariant=Sum_PID  TsampFilterVariant=InternalTs  TsampNgainVariant=Passthrough  TsampIntegralVariant=Passthrough  ExternalSaturationOutDataTypeStr=Inherit: Same as second input
      settings: SourceProductBaseCode=SL
  cfblk5 : DotProduct  OutDataTypeStr=Inherit: Inherit via internal rule
  cfblk6 : Math  Operator=conj
  cfblk7 : Product  Inputs=*
  cfblk8 : Rounding
  cfblk9 : simulink/Math Operations/MinMax Running Resettable  Function=min  vinit=0.0
  cfblk2 : Outport
  wires:
  cfblk11/1 -> cfblk8/1
  cfblk4/1 -> cfblk6/1, cfblk5/2
  cfblk7/1 -> cfblk4/1
  cfblk8/1 -> cfblk9/1
  cfblk10/1 -> cfblk9/2
  cfblk1/1 -> cfblk10/2
  cfblk9/1 -> cfblk7/1, cfblk2/1
  cfblk3/1 -> cfblk13/1, cfblk14/1
  cfblk5/1 -> cfblk3/1
  cfblk6/1 -> cfblk12/1
  cfblk12/1 -> cfblk10/1
  cfblk13/1 -> cfblk4/2
  cfblk14/1 -> cfblk5/1

== system sampleModel1739/cfblk31/cfblk10 ==
  cfblk1 : Inport
  cfblk12 : Inport  Port=2
  cfblk13 : Inport  Port=3
  cfblk10 : Assignment  DiagnosticForDimensions=Warning  IndexOptions=Index vector (dialog)  Indices=1  OutputSizes=1
  cfblk11 : simulink/Math Operations/Slider Gain  gain=1  low=0  high=2
  cfblk14 : Delay  SampleTime=1
  cfblk15 : Delay  SampleTime=1
  cfblk3 : Delay  ShowEnablePort=on  SampleTime=1
      settings: InputPortMap=u0,e6
  cfblk4 : simulink/Discrete/Difference  ICPrevInput=0.0  OutMin=[]  OutMax=[]  OutDataTypeStr=Inherit: Inherit via back propagation  OutDataType=fixdt(1, 16)  OutScaling=2^-10  DoSatur=off
  cfblk5 : DiscreteZeroPole  Poles=[0 0.5]  Gain=1
  cfblk6 : simulink/Discrete/Transfer Fcn Lead or Lag  PoleZ=0.95  ZeroZ=0.75  ICPrevOutput=0.0  ICPrevInput=0.0  DoSatur=off
      settings: SourceProductBaseCode=SL
  cfblk7 : DiscreteStateSpace
  cfblk8 : Abs  SaturateOnIntegerOverflow=off
  cfblk9 : Sum  Inputs=+-
  cfblk2 : Outport
  wires:
  cfblk11/1 -> cfblk4/1
  cfblk3/1 -> cfblk5/1, cfblk14/1
  cfblk4/1 -> cfblk9/1
  cfblk5/1 -> cfblk2/1
  cfblk7/1 -> cfblk3/1
  cfblk13/1 -> cfblk7/1
  cfblk12/1 -> cfblk10/1
  cfblk9/1 -> cfblk6/1
  cfblk1/1 -> cfblk11/1
  cfblk6/1 -> cfblk3/2
  cfblk8/1 -> cfblk10/2
  cfblk14/1 -> cfblk9/2
  cfblk10/1 -> cfblk15/1
  cfblk15/1 -> cfblk8/1

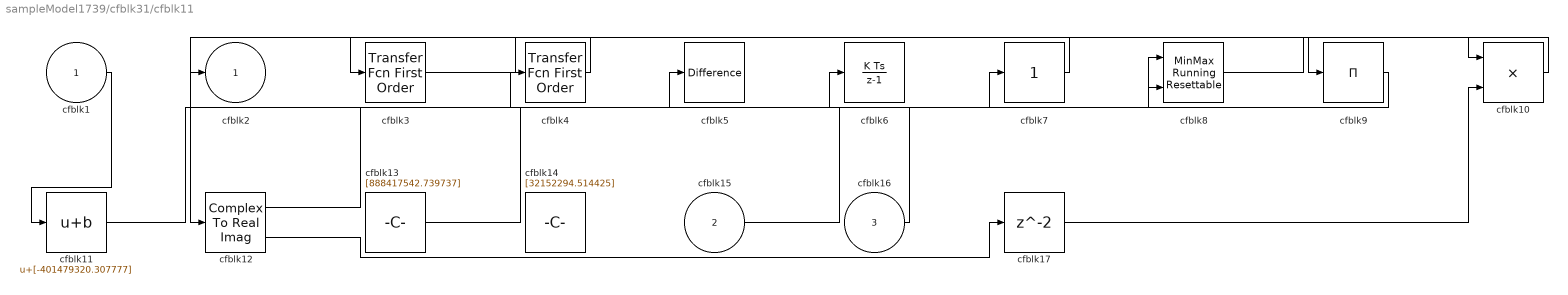
== system sampleModel1739/cfblk31/cfblk11 ==
  cfblk1 : Inport
  cfblk15 : Inport  Port=2
  cfblk16 : Inport  Port=3
  cfblk10 : Product
  cfblk11 : Bias  Bias=[-401479320.307777]  SaturateOnIntegerOverflow=off
  cfblk12 : ComplexToRealImag
  cfblk13 : Constant  Value=[888417542.739737]  SampleTime=1
  cfblk14 : Constant  Value=[32152294.514425]  SampleTime=1
  cfblk17 : Delay  SampleTime=1
  cfblk3 : simulink/Discrete/Transfer Fcn First Order  PoleZ=0.95  ICPrevOutput=0.0  DoSatur=off
  cfblk4 : simulink/Discrete/Transfer Fcn First Order  PoleZ=0.95  ICPrevOutput=0.0  DoSatur=off
  cfblk5 : simulink/Discrete/Difference  ICPrevInput=0.0  OutMin=[]  OutMax=[]  OutDataTypeStr=Inherit: Inherit via back propagation  OutDataType=fixdt(1, 16)  OutScaling=2^-10  DoSatur=off
  cfblk6 : DiscreteIntegrator  ICPrevOutput=DiscIntNeverNeededParam  ICPrevScaledInput=DiscIntNeverNeededParam
  cfblk7 : simulink/Math Operations/Slider Gain  gain=1  low=0  high=2
  cfblk8 : simulink/Math Operations/MinMax Running Resettable  Function=min  vinit=0.0
  cfblk9 : Product  Inputs=*
  cfblk2 : Outport
  wires:
  cfblk15/1 -> cfblk8/1
  cfblk13/1 -> cfblk6/1
  cfblk10/1 -> cfblk12/1
  cfblk3/1 -> cfblk9/1
  cfblk16/1 -> cfblk4/1
  cfblk4/1 -> cfblk3/1
  cfblk7/1 -> cfblk2/1
  cfblk9/1 -> cfblk8/2
  cfblk11/1 -> cfblk5/1
  cfblk8/1 -> cfblk10/1
  cfblk1/1 -> cfblk11/1
  cfblk12/1 -> cfblk7/1
  cfblk12/2 -> cfblk17/1
  cfblk17/1 -> cfblk10/2

== system sampleModel1739/cfblk31/cfblk12 ==
  cfblk1 : Inport
  cfblk9 : Inport  Port=2
  cfblk10 : Inport  Port=3
  cfblk3 : simulink/Discrete/Tapped Delay  vinit=0.0  samptime=-1  NumDelays=1  DelayOrder=Oldest  includeCurrent=off
  cfblk4 : Abs  SaturateOnIntegerOverflow=off
  cfblk5 : Math  Operator=square
  cfblk6 : Signum
  cfblk7 : Sum  Inputs=--
  cfblk8 : Constant  Value=[-697200620.604912]  SampleTime=1
  cfblk2 : Outport
  cfblk11 : Outport  Port=2
  cfblk12 : Outport  Port=3
  cfblk13 : Outport  Port=4
  cfblk14 : Outport  Port=5
  wires:
  cfblk6/1 -> cfblk12/1
  cfblk3/1 -> cfblk4/1
  cfblk8/1 -> cfblk3/1, cfblk14/1
  cfblk5/1 -> cfblk11/1
  cfblk1/1 -> cfblk2/1, cfblk6/1
  cfblk10/1 -> cfblk7/1
  cfblk4/1 -> cfblk5/1
  cfblk7/1 -> cfblk13/1
  cfblk9/1 -> cfblk7/2

== system sampleModel1739/cfblk31/cfblk13 ==
  cfblk1 : Inport
  cfblk10 : Inport  Port=2
  cfblk11 : Inport  Port=3
  cfblk13 : Delay  SampleTime=1
  cfblk3 : DiscreteFir  SampleTime=1
  cfblk4 : simulink/Math Operations/Slider Gain  gain=1  low=0  high=2
  cfblk5 : Sum  Inputs=+-
  cfblk6 : PermuteDimensions
  cfblk7 : Sum  Inputs=+-
  cfblk8 : Constant  Value=[-381651457.196367]  SampleTime=1
  cfblk9 : Constant  Value=[461964997.437330]  SampleTime=1
  cfblk2 : Outport
  cfblk12 : Outport  Port=2
  wires:
  cfblk9/1 -> cfblk3/1
  cfblk1/1 -> cfblk12/1
  cfblk3/1 -> cfblk7/1
  cfblk4/1 -> cfblk5/1
  cfblk7/1 -> cfblk6/1
  cfblk8/1 -> cfblk4/1
  cfblk11/1 -> cfblk2/1
  cfblk10/1 -> cfblk5/2
  cfblk6/1 -> cfblk13/1
  cfblk13/1 -> cfblk7/2

== system sampleModel1739/cfblk31/cfblk8 ==
  cfblk1 : Inport
  cfblk9 : Inport  Port=2
  cfblk10 : Inport  Port=3
  cfblk3 : Delay  DelayLengthSource=Input port  SampleTime=1
      settings: InputPortMap=u0,p1
  cfblk4 : DiscreteIntegrator  ICPrevOutput=DiscIntNeverNeededParam  ICPrevScaledInput=DiscIntNeverNeededParam
  cfblk5 : Delay  ShowEnablePort=on  SampleTime=1
      settings: InputPortMap=u0,e6
  cfblk6 : Constant  Value=[159511012.901454]  SampleTime=1
  cfblk7 : Constant  Value=[877393719.480230]  SampleTime=1
  cfblk8 : Constant  Value=[-943945452.438423]  SampleTime=1
  cfblk2 : Outport
  wires:
  cfblk10/1 -> cfblk3/1
  cfblk5/1 -> cfblk3/2
  cfblk3/1 -> cfblk2/1
  cfblk6/1 -> cfblk4/1
  cfblk9/1 -> cfblk5/1
  cfblk1/1 -> cfblk5/2
